simulink model "example_rzr"  (R2023b)
settings: Solver=VariableStepAuto  StartTime=0.0  StopTime=inf  RelTol=1e-3
undefined symbols (not defined in the file or in its folder): gray
settings Model: Creator=tsamak  LastModifiedBy=tsamak
settings OptimizationCC: ZeroExternalMemoryAtStartup=off  ZeroInternalMemoryAtStartup=off  InitFltsAndDblsToZero=on
settings DebuggingCC: UnderSpecifiedDimensionMsg=warning
settings HardwareCC: ProdLongLongMode=on  TargetLongLongMode=on
settings SFSimCC: SimTargetLang=C++  GPUAcceleration=on  SimDLTargetLibrary=cudnn
settings RTWCC: TargetLang=C++  GenerateGPUCode=CUDA
settings GRTTargetCC: TargetLangStandard=C++11 (ISO)  CodeInterfacePackaging=C++ class

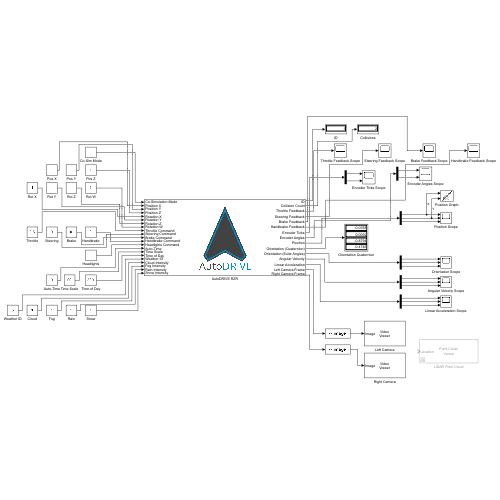
[thumbnail: Simulink's stored preview of the top-level diagram]
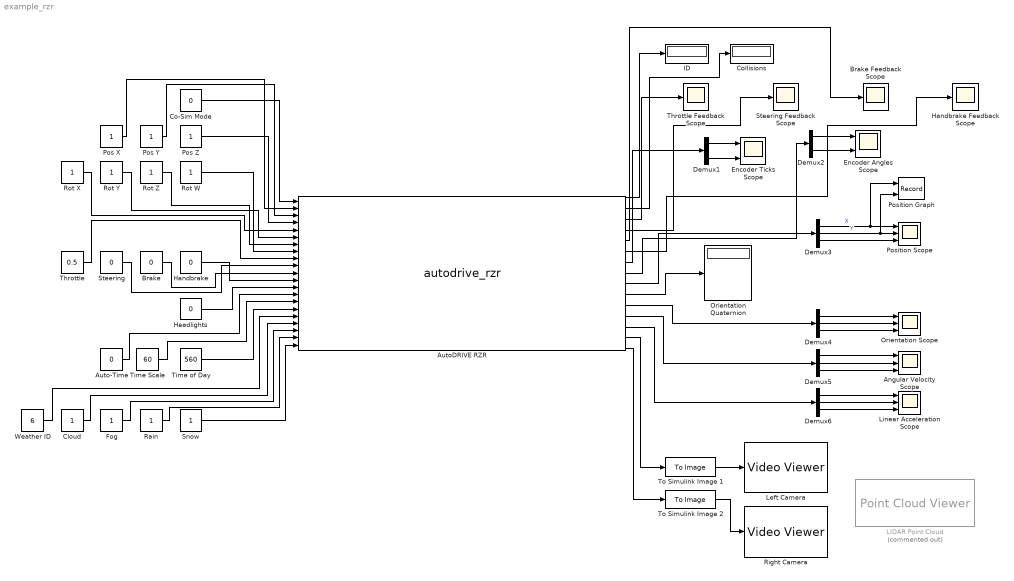
== system example_rzr ==
  Angular Velocity Scope : Scope  NumInputPorts=3
  Auto-Time : Constant  Value=0  OutDataTypeStr=boolean
  AutoDRIVE RZR : M-S-Function  FunctionName=autodrive_rzr  Parameters=Port  mask{Port=4567}
      mask Display:
      | image('autodrive_logo.png');
      | port_label('input', 1, 'Co-Simulation Mode');
      | port_label('input', 2, 'Position X');
      | port_label('input', 3, 'Position Y');
      | port_label('input', 4, 'Position Z');
      | port_label('input', 5, 'Rotation X');
      | port_label('input', 6, 'Rotation Y');
      | port_label('input', 7, 'Rotation Z');
      | port_label('input', 8, 'Rotation W');
      | port_label('input', 9, 'Throttle Command');
      | port_label('input', 10, 'Steering Command');
      | port_label('input', 11, 'Brake Command');
      | port_label('input', 12, 'Handbrake Command');
      | port_label('input', 13, 'Headlights Command');
      | port_label('input', 14, 'Auto-Time');
      | port_label('input', 15, 'Time Scale');
      | port_label('input', 16, 'Time of Day');
      | port_label('input', 17, 'Weather ID');
      | port_label('input', 18, 'Cloud Intensity');
      | port_label('input', 19, 'Fog Intensity');
      | port_label('input', 20, 'Rain Intensity');
      | port_label('input', 21, 'Snow Intensity');
      | port_label('output', 1, 'ID');
      | port_label('output', 2, 'Collision Count');
      | port_label('output', 3, 'Throttle Feedback');
      | port_label('output', 4, 'Steering Feedback');
      | port_label('output', 5, 'Brake Feedback');
      | port_label('output', 6, 'Handbrake Feedback');
      | port_label('output', 7, 'Encoder Ticks');
      | port_label('output', 8, 'Encoder Angles');
      | port_label('output', 9, 'Position');
      | port_label('output', 10, 'Orientation (Quaternion)');
      | port_label('output', 11, 'Orientation (Euler Angles)');
      | port_label('output', 12, 'Angular Velocity');
      | port_label('output', 13, 'Linear Acceleration');
      | port_label('output', 14, 'Left Camera Frame');
      | port_label('output', 15, 'Right Camera Frame');
  Brake : Constant  Value=0
  Brake Feedback Scope : Scope
  Cloud : Constant
  Co-Sim Mode : Constant  Value=0  OutDataTypeStr=uint8
  Collisions : Display
  Demux1 : Demux  Outputs=2
  Demux2 : Demux  Outputs=2
  Demux{3..6} (4 alike) : Demux  Outputs=3
  Encoder Angles Scope : Scope  NumInputPorts=2
  Encoder Ticks Scope : Scope  NumInputPorts=2
  Fog : Constant
  Handbrake : Constant  Value=0
  Handbrake Feedback Scope : Scope
  Headlights : Constant  Value=0  OutDataTypeStr=uint8
  ID : Display
  LIDAR Point Cloud : PointCloudViewer  Commented=on  FigPos=[843.666666666667 412 469.333333333333 328.666666666667]
  Left Camera : VideoViewer  colormapValue=gray(256)  FigPos=[11 410 408 304]
  Linear Acceleration Scope : Scope  NumInputPorts=3
  Orientation Quaternion : Display
  Orientation Scope : Scope  NumInputPorts=3
  Pos X : Constant
  Pos Y : Constant
  Pos Z : Constant
  Position Graph : Record  FileSettingsInternal="{\"entries\":[{\"content\":{\"excelSettings\":{\"content\":{},\"type\":\"Streamout.ExcelSettings\"}},\"type\":\"Streamout.FileSettingStorage\",\"uuid\":\"\"}],\"packageUris\":[\"http:\\/\\/schema.mathworks.com\\/mf0\\/streamout_blocks\\/R2020a\"],\"version\":\"1.0\"}"  Layout=[1 1]  SignalsInternal="{\"entries\":[{\"content\":{\"signals\":[{\"content\":{\"blockPath\":[],\"dimensions\":[1,1],\"domain\":\"\",\"lineColor\":\"#139fff\",\"plots\":[ 1 ],\"port\":1,\"sid\":[\"\"],\"signalID\":1,\"signalName\":\"X\"},\"type\":\"RecordBlkView.Signal\",\"uuid\":\"\"},{\"content\":{\"blockPath\":[],\"dimensions\":[1,1],\"domain\":\"\",\"lineColor\":\"#139fff\",\"plots\":[ 1 ],\"port\":2,\"sid\":[\"\"],\"signalID\":2,\"signalName\":\"Y\"},\"type\":\"RecordBlkView.Signal\",\"uuid\":\"\"}]},\"type\":\"RecordBlkView.InputSignals\",\"uuid\":\"\"}],\"packageUris\":[\"http:\\/\\/schema.mathworks.com\\/mf0\\/streamout_blocks\\/R2020a\"],\"version\":\"1.0\"}"  VisualizationBindings="{\"xyplotplugin\":{\"info\":[{\"series\":[{\"bindingParametersList\":[{\"parameter\":\"X-Axis\",\"signalID\":1,\"signalName\":\"X\"},{\"parameter\":\"Y-Axis\",\"signalID\":2,\"signalName\":\"Y\"}],\"seriesID\":0}],\"subplotID\":1}]}}"  CompatibilityTag=XY
  Position Scope : Scope  NumInputPorts=3
  Rain : Constant
  Right Camera : VideoViewer  colormapValue=gray(256)  FigPos=[423 410 418 304]
  Rot W : Constant
  Rot X : Constant
  Rot Y : Constant
  Rot Z : Constant
  Snow : Constant
  Steering : Constant  Value=0
  Steering Feedback Scope : Scope
  Throttle : Constant  Value=0.5
  Throttle Feedback Scope : Scope
  Time Scale : Constant  Value=60
  Time of Day : Constant  Value=560
  To Simulink Image 1 : ToImage
  To Simulink Image 2 : ToImage
  Weather ID : Constant  Value=6  OutDataTypeStr=uint8
  wires:
  Throttle/1 -> AutoDRIVE RZR/9
  Steering/1 -> AutoDRIVE RZR/10
  Demux3/2 -> Position Scope/2, Position Graph/2  "Y"
  Demux3/1 -> Position Scope/1, Position Graph/1  "X"
  Demux3/3 -> Position Scope/3
  AutoDRIVE RZR/15 -> To Simulink Image 2/1
  To Simulink Image 1/1 -> Left Camera/1
  To Simulink Image 2/1 -> Right Camera/1
  AutoDRIVE RZR/9 -> Demux3/1
  AutoDRIVE RZR/1 -> ID/1
  AutoDRIVE RZR/3 -> Throttle Feedback Scope/1
  AutoDRIVE RZR/4 -> Steering Feedback Scope/1
  AutoDRIVE RZR/7 -> Demux1/1
  Demux1/1 -> Encoder Ticks Scope/1
  Demux1/2 -> Encoder Ticks Scope/2
  Demux2/1 -> Encoder Angles Scope/1
  Demux2/2 -> Encoder Angles Scope/2
  AutoDRIVE RZR/8 -> Demux2/1
  Demux4/3 -> Orientation Scope/3
  Demux5/3 -> Angular Velocity Scope/3
  Demux6/3 -> Linear Acceleration Scope/3
  AutoDRIVE RZR/10 -> Orientation Quaternion/1
  AutoDRIVE RZR/11 -> Demux4/1
  AutoDRIVE RZR/12 -> Demux5/1
  AutoDRIVE RZR/13 -> Demux6/1
  Demux4/1 -> Orientation Scope/1
  Demux4/2 -> Orientation Scope/2
  Demux5/1 -> Angular Velocity Scope/1
  Demux5/2 -> Angular Velocity Scope/2
  Demux6/1 -> Linear Acceleration Scope/1
  Demux6/2 -> Linear Acceleration Scope/2
  Rot W/1 -> AutoDRIVE RZR/8
  Rot Z/1 -> AutoDRIVE RZR/7
  Rot Y/1 -> AutoDRIVE RZR/6
  Rot X/1 -> AutoDRIVE RZR/5
  Pos Z/1 -> AutoDRIVE RZR/4
  Pos Y/1 -> AutoDRIVE RZR/3
  Pos X/1 -> AutoDRIVE RZR/2
  Co-Sim Mode/1 -> AutoDRIVE RZR/1
  AutoDRIVE RZR/14 -> To Simulink Image 1/1
  Brake/1 -> AutoDRIVE RZR/11
  Handbrake/1 -> AutoDRIVE RZR/12
  Auto-Time/1 -> AutoDRIVE RZR/14
  Rain/1 -> AutoDRIVE RZR/20
  Fog/1 -> AutoDRIVE RZR/19
  Cloud/1 -> AutoDRIVE RZR/18
  Snow/1 -> AutoDRIVE RZR/21
  Weather ID/1 -> AutoDRIVE RZR/17
  Time Scale/1 -> AutoDRIVE RZR/15
  Time of Day/1 -> AutoDRIVE RZR/16
  Headlights/1 -> AutoDRIVE RZR/13
  AutoDRIVE RZR/2 -> Collisions/1
  AutoDRIVE RZR/5 -> Brake Feedback Scope/1
  AutoDRIVE RZR/6 -> Handbrake Feedback Scope/1
